simulink model "gm_parallel_lht_vnl"  (R2019b)
settings: Solver=FixedStepDiscrete  StartTime=0.0  StopTime=inf  RelTol=1e-3
undefined symbols (not defined in the file or in its folder): bt, height, nTheta, width
libraries: hdlsllib x199, simulink x27, hdlmdlgenlib x7, dspsrcs4 x1
(part 12 of 19)

== system gm_parallel_lht_vnl/Parallel LHT/Parallel LHT Accumulator/Accumulator with Switches/Accumulator_instance86/Block RAM ==
  wr_data : Inport  OutDataTypeStr=fixdt(0, 9, 0)  PortDimensions=1  SampleTime=6.66666666666667e-09
  wr_addr : Inport  Port=2  OutDataTypeStr=fixdt(0, 9, 0)  PortDimensions=1  SampleTime=6.66666666666667e-09
  wr_en : Inport  Port=3  OutDataTypeStr=boolean  PortDimensions=1  SampleTime=6.66666666666667e-09
  rd_addr : Inport  Port=4  OutDataTypeStr=fixdt(0, 9, 0)  PortDimensions=1  SampleTime=6.66666666666667e-09
  Simple Dual Port RAM : Subsystem
  rd_data : Outport
  wires:
  Simple Dual Port RAM/1(rd_data) -> rd_data/1
  wr_data/1 -> Simple Dual Port RAM/1(wr_data)
  wr_addr/1 -> Simple Dual Port RAM/2(wr_addr)
  wr_en/1 -> Simple Dual Port RAM/3(wr_en)
  rd_addr/1 -> Simple Dual Port RAM/4(rd_addr)

== system gm_parallel_lht_vnl/Parallel LHT/Parallel LHT Accumulator/Accumulator with Switches/Accumulator_instance87/Block RAM ==
  wr_data : Inport  OutDataTypeStr=fixdt(0, 9, 0)  PortDimensions=1  SampleTime=6.66666666666667e-09
  wr_addr : Inport  Port=2  OutDataTypeStr=fixdt(0, 9, 0)  PortDimensions=1  SampleTime=6.66666666666667e-09
  wr_en : Inport  Port=3  OutDataTypeStr=boolean  PortDimensions=1  SampleTime=6.66666666666667e-09
  rd_addr : Inport  Port=4  OutDataTypeStr=fixdt(0, 9, 0)  PortDimensions=1  SampleTime=6.66666666666667e-09
  Simple Dual Port RAM : Subsystem
  rd_data : Outport
  wires:
  Simple Dual Port RAM/1(rd_data) -> rd_data/1
  wr_data/1 -> Simple Dual Port RAM/1(wr_data)
  wr_addr/1 -> Simple Dual Port RAM/2(wr_addr)
  wr_en/1 -> Simple Dual Port RAM/3(wr_en)
  rd_addr/1 -> Simple Dual Port RAM/4(rd_addr)

== system gm_parallel_lht_vnl/Parallel LHT/Parallel LHT Accumulator/Accumulator with Switches/Accumulator_instance88/Block RAM ==
  wr_data : Inport  OutDataTypeStr=fixdt(0, 9, 0)  PortDimensions=1  SampleTime=6.66666666666667e-09
  wr_addr : Inport  Port=2  OutDataTypeStr=fixdt(0, 9, 0)  PortDimensions=1  SampleTime=6.66666666666667e-09
  wr_en : Inport  Port=3  OutDataTypeStr=boolean  PortDimensions=1  SampleTime=6.66666666666667e-09
  rd_addr : Inport  Port=4  OutDataTypeStr=fixdt(0, 9, 0)  PortDimensions=1  SampleTime=6.66666666666667e-09
  Simple Dual Port RAM : Subsystem
  rd_data : Outport
  wires:
  Simple Dual Port RAM/1(rd_data) -> rd_data/1
  wr_data/1 -> Simple Dual Port RAM/1(wr_data)
  wr_addr/1 -> Simple Dual Port RAM/2(wr_addr)
  wr_en/1 -> Simple Dual Port RAM/3(wr_en)
  rd_addr/1 -> Simple Dual Port RAM/4(rd_addr)

== system gm_parallel_lht_vnl/Parallel LHT/Parallel LHT Accumulator/Accumulator with Switches/Accumulator_instance89/Block RAM ==
  wr_data : Inport  OutDataTypeStr=fixdt(0, 9, 0)  PortDimensions=1  SampleTime=6.66666666666667e-09
  wr_addr : Inport  Port=2  OutDataTypeStr=fixdt(0, 9, 0)  PortDimensions=1  SampleTime=6.66666666666667e-09
  wr_en : Inport  Port=3  OutDataTypeStr=boolean  PortDimensions=1  SampleTime=6.66666666666667e-09
  rd_addr : Inport  Port=4  OutDataTypeStr=fixdt(0, 9, 0)  PortDimensions=1  SampleTime=6.66666666666667e-09
  Simple Dual Port RAM : Subsystem
  rd_data : Outport
  wires:
  Simple Dual Port RAM/1(rd_data) -> rd_data/1
  wr_data/1 -> Simple Dual Port RAM/1(wr_data)
  wr_addr/1 -> Simple Dual Port RAM/2(wr_addr)
  wr_en/1 -> Simple Dual Port RAM/3(wr_en)
  rd_addr/1 -> Simple Dual Port RAM/4(rd_addr)

== system gm_parallel_lht_vnl/Parallel LHT/Parallel LHT Accumulator/Accumulator with Switches/Accumulator_instance9/Block RAM ==
  wr_data : Inport  OutDataTypeStr=fixdt(0, 9, 0)  PortDimensions=1  SampleTime=6.66666666666667e-09
  wr_addr : Inport  Port=2  OutDataTypeStr=fixdt(0, 9, 0)  PortDimensions=1  SampleTime=6.66666666666667e-09
  wr_en : Inport  Port=3  OutDataTypeStr=boolean  PortDimensions=1  SampleTime=6.66666666666667e-09
  rd_addr : Inport  Port=4  OutDataTypeStr=fixdt(0, 9, 0)  PortDimensions=1  SampleTime=6.66666666666667e-09
  Simple Dual Port RAM : Subsystem
  rd_data : Outport
  wires:
  Simple Dual Port RAM/1(rd_data) -> rd_data/1
  wr_data/1 -> Simple Dual Port RAM/1(wr_data)
  wr_addr/1 -> Simple Dual Port RAM/2(wr_addr)
  wr_en/1 -> Simple Dual Port RAM/3(wr_en)
  rd_addr/1 -> Simple Dual Port RAM/4(rd_addr)

== system gm_parallel_lht_vnl/Parallel LHT/Parallel LHT Accumulator/Accumulator with Switches/Accumulator_instance90/Block RAM ==
  wr_data : Inport  OutDataTypeStr=fixdt(0, 9, 0)  PortDimensions=1  SampleTime=6.66666666666667e-09
  wr_addr : Inport  Port=2  OutDataTypeStr=fixdt(0, 9, 0)  PortDimensions=1  SampleTime=6.66666666666667e-09
  wr_en : Inport  Port=3  OutDataTypeStr=boolean  PortDimensions=1  SampleTime=6.66666666666667e-09
  rd_addr : Inport  Port=4  OutDataTypeStr=fixdt(0, 9, 0)  PortDimensions=1  SampleTime=6.66666666666667e-09
  Simple Dual Port RAM : Subsystem
  rd_data : Outport
  wires:
  Simple Dual Port RAM/1(rd_data) -> rd_data/1
  wr_data/1 -> Simple Dual Port RAM/1(wr_data)
  wr_addr/1 -> Simple Dual Port RAM/2(wr_addr)
  wr_en/1 -> Simple Dual Port RAM/3(wr_en)
  rd_addr/1 -> Simple Dual Port RAM/4(rd_addr)

== system gm_parallel_lht_vnl/Parallel LHT/Parallel LHT Accumulator/Accumulator with Switches/Accumulator_instance91/Block RAM ==
  wr_data : Inport  OutDataTypeStr=fixdt(0, 9, 0)  PortDimensions=1  SampleTime=6.66666666666667e-09
  wr_addr : Inport  Port=2  OutDataTypeStr=fixdt(0, 9, 0)  PortDimensions=1  SampleTime=6.66666666666667e-09
  wr_en : Inport  Port=3  OutDataTypeStr=boolean  PortDimensions=1  SampleTime=6.66666666666667e-09
  rd_addr : Inport  Port=4  OutDataTypeStr=fixdt(0, 9, 0)  PortDimensions=1  SampleTime=6.66666666666667e-09
  Simple Dual Port RAM : Subsystem
  rd_data : Outport
  wires:
  Simple Dual Port RAM/1(rd_data) -> rd_data/1
  wr_data/1 -> Simple Dual Port RAM/1(wr_data)
  wr_addr/1 -> Simple Dual Port RAM/2(wr_addr)
  wr_en/1 -> Simple Dual Port RAM/3(wr_en)
  rd_addr/1 -> Simple Dual Port RAM/4(rd_addr)

== system gm_parallel_lht_vnl/Parallel LHT/Parallel LHT Accumulator/Accumulator with Switches/Accumulator_instance92/Block RAM ==
  wr_data : Inport  OutDataTypeStr=fixdt(0, 9, 0)  PortDimensions=1  SampleTime=6.66666666666667e-09
  wr_addr : Inport  Port=2  OutDataTypeStr=fixdt(0, 9, 0)  PortDimensions=1  SampleTime=6.66666666666667e-09
  wr_en : Inport  Port=3  OutDataTypeStr=boolean  PortDimensions=1  SampleTime=6.66666666666667e-09
  rd_addr : Inport  Port=4  OutDataTypeStr=fixdt(0, 9, 0)  PortDimensions=1  SampleTime=6.66666666666667e-09
  Simple Dual Port RAM : Subsystem
  rd_data : Outport
  wires:
  Simple Dual Port RAM/1(rd_data) -> rd_data/1
  wr_data/1 -> Simple Dual Port RAM/1(wr_data)
  wr_addr/1 -> Simple Dual Port RAM/2(wr_addr)
  wr_en/1 -> Simple Dual Port RAM/3(wr_en)
  rd_addr/1 -> Simple Dual Port RAM/4(rd_addr)

== system gm_parallel_lht_vnl/Parallel LHT/Parallel LHT Accumulator/Accumulator with Switches/Accumulator_instance93/Block RAM ==
  wr_data : Inport  OutDataTypeStr=fixdt(0, 9, 0)  PortDimensions=1  SampleTime=6.66666666666667e-09
  wr_addr : Inport  Port=2  OutDataTypeStr=fixdt(0, 9, 0)  PortDimensions=1  SampleTime=6.66666666666667e-09
  wr_en : Inport  Port=3  OutDataTypeStr=boolean  PortDimensions=1  SampleTime=6.66666666666667e-09
  rd_addr : Inport  Port=4  OutDataTypeStr=fixdt(0, 9, 0)  PortDimensions=1  SampleTime=6.66666666666667e-09
  Simple Dual Port RAM : Subsystem
  rd_data : Outport
  wires:
  Simple Dual Port RAM/1(rd_data) -> rd_data/1
  wr_data/1 -> Simple Dual Port RAM/1(wr_data)
  wr_addr/1 -> Simple Dual Port RAM/2(wr_addr)
  wr_en/1 -> Simple Dual Port RAM/3(wr_en)
  rd_addr/1 -> Simple Dual Port RAM/4(rd_addr)

== system gm_parallel_lht_vnl/Parallel LHT/Parallel LHT Accumulator/Accumulator with Switches/Accumulator_instance94/Block RAM ==
  wr_data : Inport  OutDataTypeStr=fixdt(0, 9, 0)  PortDimensions=1  SampleTime=6.66666666666667e-09
  wr_addr : Inport  Port=2  OutDataTypeStr=fixdt(0, 9, 0)  PortDimensions=1  SampleTime=6.66666666666667e-09
  wr_en : Inport  Port=3  OutDataTypeStr=boolean  PortDimensions=1  SampleTime=6.66666666666667e-09
  rd_addr : Inport  Port=4  OutDataTypeStr=fixdt(0, 9, 0)  PortDimensions=1  SampleTime=6.66666666666667e-09
  Simple Dual Port RAM : Subsystem
  rd_data : Outport
  wires:
  Simple Dual Port RAM/1(rd_data) -> rd_data/1
  wr_data/1 -> Simple Dual Port RAM/1(wr_data)
  wr_addr/1 -> Simple Dual Port RAM/2(wr_addr)
  wr_en/1 -> Simple Dual Port RAM/3(wr_en)
  rd_addr/1 -> Simple Dual Port RAM/4(rd_addr)

== system gm_parallel_lht_vnl/Parallel LHT/Parallel LHT Accumulator/Accumulator with Switches/Accumulator_instance95/Block RAM ==
  wr_data : Inport  OutDataTypeStr=fixdt(0, 9, 0)  PortDimensions=1  SampleTime=6.66666666666667e-09
  wr_addr : Inport  Port=2  OutDataTypeStr=fixdt(0, 9, 0)  PortDimensions=1  SampleTime=6.66666666666667e-09
  wr_en : Inport  Port=3  OutDataTypeStr=boolean  PortDimensions=1  SampleTime=6.66666666666667e-09
  rd_addr : Inport  Port=4  OutDataTypeStr=fixdt(0, 9, 0)  PortDimensions=1  SampleTime=6.66666666666667e-09
  Simple Dual Port RAM : Subsystem
  rd_data : Outport
  wires:
  Simple Dual Port RAM/1(rd_data) -> rd_data/1
  wr_data/1 -> Simple Dual Port RAM/1(wr_data)
  wr_addr/1 -> Simple Dual Port RAM/2(wr_addr)
  wr_en/1 -> Simple Dual Port RAM/3(wr_en)
  rd_addr/1 -> Simple Dual Port RAM/4(rd_addr)

== system gm_parallel_lht_vnl/Parallel LHT/Parallel LHT Accumulator/Accumulator with Switches/Accumulator_instance96/Block RAM ==
  wr_data : Inport  OutDataTypeStr=fixdt(0, 9, 0)  PortDimensions=1  SampleTime=6.66666666666667e-09
  wr_addr : Inport  Port=2  OutDataTypeStr=fixdt(0, 9, 0)  PortDimensions=1  SampleTime=6.66666666666667e-09
  wr_en : Inport  Port=3  OutDataTypeStr=boolean  PortDimensions=1  SampleTime=6.66666666666667e-09
  rd_addr : Inport  Port=4  OutDataTypeStr=fixdt(0, 9, 0)  PortDimensions=1  SampleTime=6.66666666666667e-09
  Simple Dual Port RAM : Subsystem
  rd_data : Outport
  wires:
  Simple Dual Port RAM/1(rd_data) -> rd_data/1
  wr_data/1 -> Simple Dual Port RAM/1(wr_data)
  wr_addr/1 -> Simple Dual Port RAM/2(wr_addr)
  wr_en/1 -> Simple Dual Port RAM/3(wr_en)
  rd_addr/1 -> Simple Dual Port RAM/4(rd_addr)

== system gm_parallel_lht_vnl/Parallel LHT/Parallel LHT Accumulator/Accumulator with Switches/Accumulator_instance97/Block RAM ==
  wr_data : Inport  OutDataTypeStr=fixdt(0, 9, 0)  PortDimensions=1  SampleTime=6.66666666666667e-09
  wr_addr : Inport  Port=2  OutDataTypeStr=fixdt(0, 9, 0)  PortDimensions=1  SampleTime=6.66666666666667e-09
  wr_en : Inport  Port=3  OutDataTypeStr=boolean  PortDimensions=1  SampleTime=6.66666666666667e-09
  rd_addr : Inport  Port=4  OutDataTypeStr=fixdt(0, 9, 0)  PortDimensions=1  SampleTime=6.66666666666667e-09
  Simple Dual Port RAM : Subsystem
  rd_data : Outport
  wires:
  Simple Dual Port RAM/1(rd_data) -> rd_data/1
  wr_data/1 -> Simple Dual Port RAM/1(wr_data)
  wr_addr/1 -> Simple Dual Port RAM/2(wr_addr)
  wr_en/1 -> Simple Dual Port RAM/3(wr_en)
  rd_addr/1 -> Simple Dual Port RAM/4(rd_addr)

== system gm_parallel_lht_vnl/Parallel LHT/Parallel LHT Accumulator/Accumulator with Switches/Accumulator_instance98/Block RAM ==
  wr_data : Inport  OutDataTypeStr=fixdt(0, 9, 0)  PortDimensions=1  SampleTime=6.66666666666667e-09
  wr_addr : Inport  Port=2  OutDataTypeStr=fixdt(0, 9, 0)  PortDimensions=1  SampleTime=6.66666666666667e-09
  wr_en : Inport  Port=3  OutDataTypeStr=boolean  PortDimensions=1  SampleTime=6.66666666666667e-09
  rd_addr : Inport  Port=4  OutDataTypeStr=fixdt(0, 9, 0)  PortDimensions=1  SampleTime=6.66666666666667e-09
  Simple Dual Port RAM : Subsystem
  rd_data : Outport
  wires:
  Simple Dual Port RAM/1(rd_data) -> rd_data/1
  wr_data/1 -> Simple Dual Port RAM/1(wr_data)
  wr_addr/1 -> Simple Dual Port RAM/2(wr_addr)
  wr_en/1 -> Simple Dual Port RAM/3(wr_en)
  rd_addr/1 -> Simple Dual Port RAM/4(rd_addr)

== system gm_parallel_lht_vnl/Parallel LHT/Parallel LHT Accumulator/Accumulator with Switches/Accumulator_instance99/Block RAM ==
  wr_data : Inport  OutDataTypeStr=fixdt(0, 9, 0)  PortDimensions=1  SampleTime=6.66666666666667e-09
  wr_addr : Inport  Port=2  OutDataTypeStr=fixdt(0, 9, 0)  PortDimensions=1  SampleTime=6.66666666666667e-09
  wr_en : Inport  Port=3  OutDataTypeStr=boolean  PortDimensions=1  SampleTime=6.66666666666667e-09
  rd_addr : Inport  Port=4  OutDataTypeStr=fixdt(0, 9, 0)  PortDimensions=1  SampleTime=6.66666666666667e-09
  Simple Dual Port RAM : Subsystem
  rd_data : Outport
  wires:
  Simple Dual Port RAM/1(rd_data) -> rd_data/1
  wr_data/1 -> Simple Dual Port RAM/1(wr_data)
  wr_addr/1 -> Simple Dual Port RAM/2(wr_addr)
  wr_en/1 -> Simple Dual Port RAM/3(wr_en)
  rd_addr/1 -> Simple Dual Port RAM/4(rd_addr)

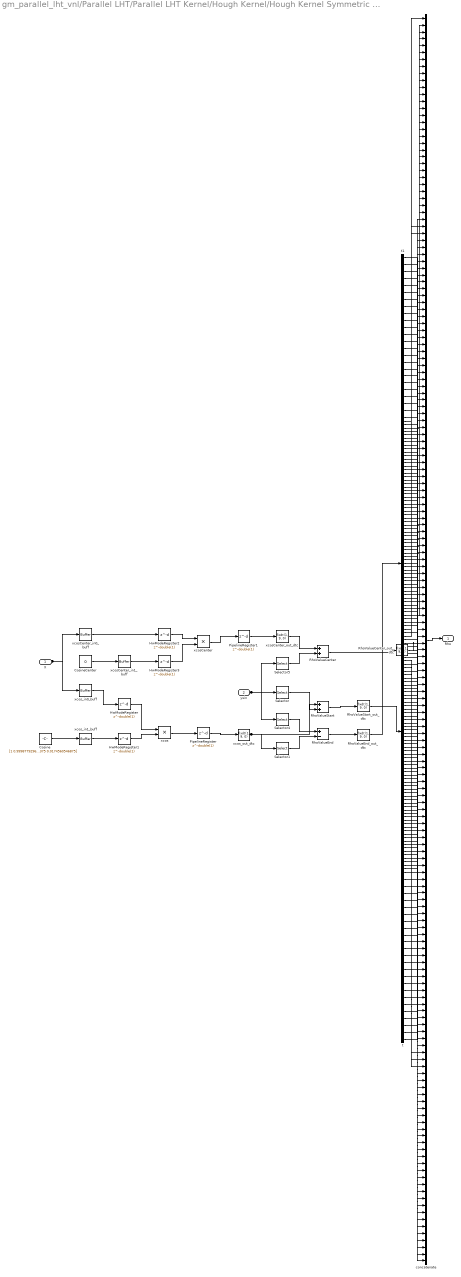
== system gm_parallel_lht_vnl/Parallel LHT/Parallel LHT Kernel/Hough Kernel/Hough Kernel Symmetric Look Ahead/Hough Kernel Symmetric ==
  X : Inport  OutDataTypeStr=fixdt(1, 9, 0)  PortDimensions=1  SampleTime=6.66666666666667e-09
  ysin : Inport  Port=2  OutDataTypeStr=int8  PortDimensions=[1 91]  SampleTime=6.66666666666667e-09
  Cosine : Constant  Value=[1 0.9998779296875 0.9993896484375 0.9986572265625 0.99755859375 0.9962158203125 0.9945068359375 0.9925537109375 0.99029541015625 0.9876708984375 0.98480224609375 0.98162841796875 0.9781494140625 0.974365234375 0.97027587890625 0.9659423828125 0.96124267578125 0.956298828125 0.9510498046875 0.94549560546875 0.939697265625 0.93359375 0.92718505859375 0.9205322265625 0.91357421875 0.90631103515625 0.8988037109375 0.8909912109375 0.8829345703125 0.8746337890625 0.86602783203125 0.857177734375 0.8480224609375 0.83868408203125 0.82904052734375 0.81915283203125 0.80902099609375 0.79864501953125 0.78802490234375 0.77716064453125 0.76605224609375 0.75469970703125 0.7431640625 0.7313232421875 0.7193603515625 0.70709228515625 0.69464111328125 0.6820068359375 0.66912841796875 0.65606689453125 0.64276123046875 0.62933349609375 0.61566162109375 0.601806640625 0.5877685546875 0.57354736328125 0.5592041015625 0.54461669921875 0.5299072265625 0.5150146484375 0.5 0.48480224609375 0.469482421875 0.4539794921875 0.4383544921875 0.422607421875 0.40673828125 0.3907470703125 0.3746337890625 0.3583984375 0.342041015625 0.3255615234375 0.30902099609375 0.2923583984375 0.275634765625 0.2587890625 0.241943359375 0.2249755859375 0.2078857421875 0.1907958984375 0.17364501953125 0.15643310546875 0.13916015625 0.12188720703125 0.10455322265625 0.087158203125 0.06976318359375 0.05230712890625 0.034912109375 0.0174560546875]  VectorParams1D=off  OutDataTypeStr=fixdt(1, 16, 14)  SampleTime=-1
  CosineCenter : Constant  Value=0  VectorParams1D=off  OutDataTypeStr=fixdt(1, 16, 14)  SampleTime=-1
  HwModeRegister{,1..3} (4 alike) : Delay  DelayLength=double(1)  InitialCondition=0  SampleTime=6.66666666666667e-09
  PipelineRegister : Delay  DelayLength=double(1)  InitialCondition=0  SampleTime=6.66666666666667e-09
  PipelineRegister1 : Delay  DelayLength=double(1)  InitialCondition=0  SampleTime=6.66666666666667e-09
  RhoValueCenter : Sum  AccumDataTypeStr=fixdt(1, 10, 0)  OutDataTypeStr=fixdt(1, 10, 0)  SampleTime=6.66666666666667e-09
  RhoValueCenter_out_dtc : DataTypeConversion  OutDataTypeStr=fixdt(1, 9, 0)  RndMeth=Round  SampleTime=6.66666666666667e-09
  RhoValueEnd : Sum  Inputs=+-  AccumDataTypeStr=fixdt(1, 10, 0)  OutDataTypeStr=fixdt(1, 10, 0)  SampleTime=6.66666666666667e-09
  RhoValueEnd_out_dtc : DataTypeConversion  OutDataTypeStr=fixdt(1, 9, 0)  RndMeth=Round  SampleTime=6.66666666666667e-09
  RhoValueStart : Sum  AccumDataTypeStr=fixdt(1, 10, 0)  OutDataTypeStr=fixdt(1, 10, 0)  SampleTime=6.66666666666667e-09
  RhoValueStart_out_dtc : DataTypeConversion  OutDataTypeStr=fixdt(1, 9, 0)  RndMeth=Round  SampleTime=6.66666666666667e-09
  Selector : Selector  NumberOfDimensions=2  IndexMode=Zero-based  SampleTime=6.66666666666667e-09  IndexOptions=Index vector (dialog),Index vector (dialog)  Indices=double(0),double([0 1 2 3 4 5 6 7 8 9 10 11 12 13 14 15 16 17 18 19 20 21 22 23 24 25 26 27 28 29 30 31 32 33 34 35 36 37 38 39 40 41 42 43 44 45 46 47 48 49 50 51 52 53 54 55 56 57 58 59 60 61 62 63 64 65 66 67 68 69 70 71 72 73 74 75 76 77 78 79 80 81 82 83 84 85 86 87 88 89])  OutputSizes=double(1),double(1)
  Selector1 : Selector  NumberOfDimensions=2  IndexMode=Zero-based  SampleTime=6.66666666666667e-09  IndexOptions=Index vector (dialog),Index vector (dialog)  Indices=double(0),double([89 88 87 86 85 84 83 82 81 80 79 78 77 76 75 74 73 72 71 70 69 68 67 66 65 64 63 62 61 60 59 58 57 56 55 54 53 52 51 50 49 48 47 46 45 44 43 42 41 40 39 38 37 36 35 34 33 32 31 30 29 28 27 26 25 24 23 22 21 20 19 18 17 16 15 14 13 12 11 10 9 8 7 6 5 4 3 2 1])  OutputSizes=double(1),double(1)
  Selector4 : Selector  NumberOfDimensions=2  IndexMode=Zero-based  SampleTime=6.66666666666667e-09  IndexOptions=Index vector (dialog),Index vector (dialog)  Indices=double(0),double([89 88 87 86 85 84 83 82 81 80 79 78 77 76 75 74 73 72 71 70 69 68 67 66 65 64 63 62 61 60 59 58 57 56 55 54 53 52 51 50 49 48 47 46 45 44 43 42 41 40 39 38 37 36 35 34 33 32 31 30 29 28 27 26 25 24 23 22 21 20 19 18 17 16 15 14 13 12 11 10 9 8 7 6 5 4 3 2 1])  OutputSizes=double(1),double(1)
  Selector5 : Selector  NumberOfDimensions=2  IndexMode=Zero-based  SampleTime=6.66666666666667e-09  IndexOptions=Index vector (dialog),Index vector (dialog)  Indices=double(0),double(90)  OutputSizes=double(1),double(1)
  concatenate : Concatenate  NumInputs=180  Mode=Multidimensional array  ConcatenateDimension=2
  t : Demux  Outputs=90
  t1 : Demux  Outputs=89
  xcos : Product  Inputs=**  OutDataTypeStr=fixdt(1, 25, 14)  SampleTime=6.66666666666667e-09
  xcosCenter : Product  Inputs=**  OutDataTypeStr=fixdt(1, 25, 14)  SampleTime=6.66666666666667e-09
  xcosCenter_in0_buff : hdlmdlgenlib/Buffer
      settings: SourceProductName=Simulink  SourceProductBaseCode=SL
  xcosCenter_in1_buff : hdlmdlgenlib/Buffer
      settings: SourceProductName=Simulink  SourceProductBaseCode=SL
  xcosCenter_out_dtc : DataTypeConversion  OutDataTypeStr=fixdt(1, 9, 0)  RndMeth=Round  SampleTime=6.66666666666667e-09
  xcos_in0_buff : hdlmdlgenlib/Buffer
      settings: SourceProductName=Simulink  SourceProductBaseCode=SL
  xcos_in1_buff : hdlmdlgenlib/Buffer
      settings: SourceProductName=Simulink  SourceProductBaseCode=SL
  xcos_out_dtc : DataTypeConversion  OutDataTypeStr=fixdt(1, 9, 0)  RndMeth=Round  SampleTime=6.66666666666667e-09
  Rho : Outport  VectorParamsAs1DForOutWhenUnconnected=off
  wires:
  xcosCenter_in1_buff/1 -> HwModeRegister3/1
  xcosCenter_in0_buff/1 -> HwModeRegister2/1
  HwModeRegister3/1 -> xcosCenter/2
  HwModeRegister2/1 -> xcosCenter/1
  xcosCenter/1 -> PipelineRegister1/1
  xcos_in1_buff/1 -> HwModeRegister1/1
  xcos_in0_buff/1 -> HwModeRegister/1
  HwModeRegister1/1 -> xcos/2
  HwModeRegister/1 -> xcos/1
  xcos/1 -> PipelineRegister/1
  t1/89 -> concatenate/180
  t1/88 -> concatenate/179
  t1/87 -> concatenate/178
  t1/86 -> concatenate/177
  t1/85 -> concatenate/176
  t1/84 -> concatenate/175
  t1/83 -> concatenate/174
  t1/82 -> concatenate/173
  t1/81 -> concatenate/172
  t1/80 -> concatenate/171
  t1/79 -> concatenate/170
  t1/78 -> concatenate/169
  t1/77 -> concatenate/168
  t1/76 -> concatenate/167
  t1/75 -> concatenate/166
  t1/74 -> concatenate/165
  t1/73 -> concatenate/164
  t1/72 -> concatenate/163
  t1/71 -> concatenate/162
  t1/70 -> concatenate/161
  t1/69 -> concatenate/160
  t1/68 -> concatenate/159
  t1/67 -> concatenate/158
  t1/66 -> concatenate/157
  t1/65 -> concatenate/156
  t1/64 -> concatenate/155
  t1/63 -> concatenate/154
  t1/62 -> concatenate/153
  t1/61 -> concatenate/152
  t1/60 -> concatenate/151
  t1/59 -> concatenate/150
  t1/58 -> concatenate/149
  t1/57 -> concatenate/148
  t1/56 -> concatenate/147
  t1/55 -> concatenate/146
  t1/54 -> concatenate/145
  t1/53 -> concatenate/144
  t1/52 -> concatenate/143
  t1/51 -> concatenate/142
  t1/50 -> concatenate/141
  t1/49 -> concatenate/140
  t1/48 -> concatenate/139
  t1/47 -> concatenate/138
  t1/46 -> concatenate/137
  t1/45 -> concatenate/136
  t1/44 -> concatenate/135
  t1/43 -> concatenate/134
  t1/42 -> concatenate/133
  t1/41 -> concatenate/132
  t1/40 -> concatenate/131
  t1/39 -> concatenate/130
  t1/38 -> concatenate/129
  t1/37 -> concatenate/128
  t1/36 -> concatenate/127
  t1/35 -> concatenate/126
  t1/34 -> concatenate/125
  t1/33 -> concatenate/124
  t1/32 -> concatenate/123
  t1/31 -> concatenate/122
  t1/30 -> concatenate/121
  t1/29 -> concatenate/120
  t1/28 -> concatenate/119
  t1/27 -> concatenate/118
  t1/26 -> concatenate/117
  t1/25 -> concatenate/116
  t1/24 -> concatenate/115
  t1/23 -> concatenate/114
  t1/22 -> concatenate/113
  t1/21 -> concatenate/112
  t1/20 -> concatenate/111
  t1/19 -> concatenate/110
  t1/18 -> concatenate/109
  t1/17 -> concatenate/108
  t1/16 -> concatenate/107
  t1/15 -> concatenate/106
  t1/14 -> concatenate/105
  t1/13 -> concatenate/104
  t1/12 -> concatenate/103
  t1/11 -> concatenate/102
  t1/10 -> concatenate/101
  t1/9 -> concatenate/100
  t1/8 -> concatenate/99
  t1/7 -> concatenate/98
  t1/6 -> concatenate/97
  t1/5 -> concatenate/96
  t1/4 -> concatenate/95
  t1/3 -> concatenate/94
  t1/2 -> concatenate/93
  t1/1 -> concatenate/92
  t/90 -> concatenate/90
  t/89 -> concatenate/89
  t/88 -> concatenate/88
  t/87 -> concatenate/87
  t/86 -> concatenate/86
  t/85 -> concatenate/85
  t/84 -> concatenate/84
  t/83 -> concatenate/83
  t/82 -> concatenate/82
  t/81 -> concatenate/81
  t/80 -> concatenate/80
  t/79 -> concatenate/79
  t/78 -> concatenate/78
  t/77 -> concatenate/77
  t/76 -> concatenate/76
  t/75 -> concatenate/75
  t/74 -> concatenate/74
  t/73 -> concatenate/73
  t/72 -> concatenate/72
  t/71 -> concatenate/71
  t/70 -> concatenate/70
  t/69 -> concatenate/69
  t/68 -> concatenate/68
  t/67 -> concatenate/67
  t/66 -> concatenate/66
  t/65 -> concatenate/65
  t/64 -> concatenate/64
  t/63 -> concatenate/63
  t/62 -> concatenate/62
  t/61 -> concatenate/61
  t/60 -> concatenate/60
  t/59 -> concatenate/59
  t/58 -> concatenate/58
  t/57 -> concatenate/57
  t/56 -> concatenate/56
  t/55 -> concatenate/55
  t/54 -> concatenate/54
  t/53 -> concatenate/53
  t/52 -> concatenate/52
  t/51 -> concatenate/51
  t/50 -> concatenate/50
  t/49 -> concatenate/49
  t/48 -> concatenate/48
  t/47 -> concatenate/47
  t/46 -> concatenate/46
  t/45 -> concatenate/45
  t/44 -> concatenate/44
  t/43 -> concatenate/43
  t/42 -> concatenate/42
  t/41 -> concatenate/41
  t/40 -> concatenate/40
  t/39 -> concatenate/39
  t/38 -> concatenate/38
  t/37 -> concatenate/37
  t/36 -> concatenate/36
  t/35 -> concatenate/35
  t/34 -> concatenate/34
  t/33 -> concatenate/33
  t/32 -> concatenate/32
  t/31 -> concatenate/31
  t/30 -> concatenate/30
  t/29 -> concatenate/29
  t/28 -> concatenate/28
  t/27 -> concatenate/27
  t/26 -> concatenate/26
  t/25 -> concatenate/25
  t/24 -> concatenate/24
  t/23 -> concatenate/23
  t/22 -> concatenate/22
  t/21 -> concatenate/21
  t/20 -> concatenate/20
  t/19 -> concatenate/19
  t/18 -> concatenate/18
  t/17 -> concatenate/17
  t/16 -> concatenate/16
  t/15 -> concatenate/15
  t/14 -> concatenate/14
  t/13 -> concatenate/13
  t/12 -> concatenate/12
  t/11 -> concatenate/11
  t/10 -> concatenate/10
  t/9 -> concatenate/9
  t/8 -> concatenate/8
  t/7 -> concatenate/7
  t/6 -> concatenate/6
  t/5 -> concatenate/5
  t/4 -> concatenate/4
  t/3 -> concatenate/3
  t/2 -> concatenate/2
  t/1 -> concatenate/1
  CosineCenter/1 -> xcosCenter_in1_buff/1
  PipelineRegister1/1 -> xcosCenter_out_dtc/1
  xcosCenter_out_dtc/1 -> RhoValueCenter/1
  RhoValueCenter/1 -> RhoValueCenter_out_dtc/1
  Selector5/1 -> RhoValueCenter/2
  RhoValueCenter_out_dtc/1 -> concatenate/91
  RhoValueStart_out_dtc/1 -> t/1
  RhoValueStart/1 -> RhoValueStart_out_dtc/1
  Selector/1 -> RhoValueStart/2
  xcos_out_dtc/1 -> RhoValueStart/1, Selector1/1
  PipelineRegister/1 -> xcos_out_dtc/1
  Selector1/1 -> RhoValueEnd/2
  RhoValueEnd/1 -> RhoValueEnd_out_dtc/1
  Selector4/1 -> RhoValueEnd/1
  RhoValueEnd_out_dtc/1 -> t1/1
  ysin/1 -> Selector5/1, Selector4/1, Selector/1
  X/1 -> xcos_in0_buff/1, xcosCenter_in0_buff/1
  concatenate/1 -> Rho/1
  Cosine/1 -> xcos_in1_buff/1
